simulink model "model_SCARA_comp_torque_joint_space"  (R2022b)
settings: Solver=VariableStepAuto  StartTime=0.0  StopTime=times_way(end)  RelTol=1e-3
undefined symbols (not defined in the file or in its folder): eta_des0, q1_0, q1_dot_0, q2_0, q2_dot_0, q3_0, q3_dot_0, q4_0, q4_dot_0
libraries: robotcorelib x1
settings Model: Creator=anton  LastModifiedBy=anton

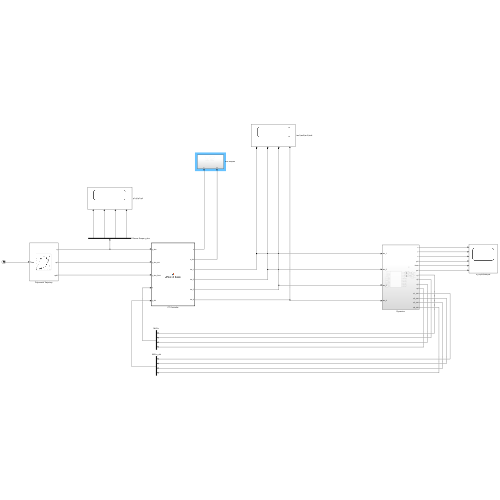
[thumbnail: Simulink's stored preview of the top-level diagram]
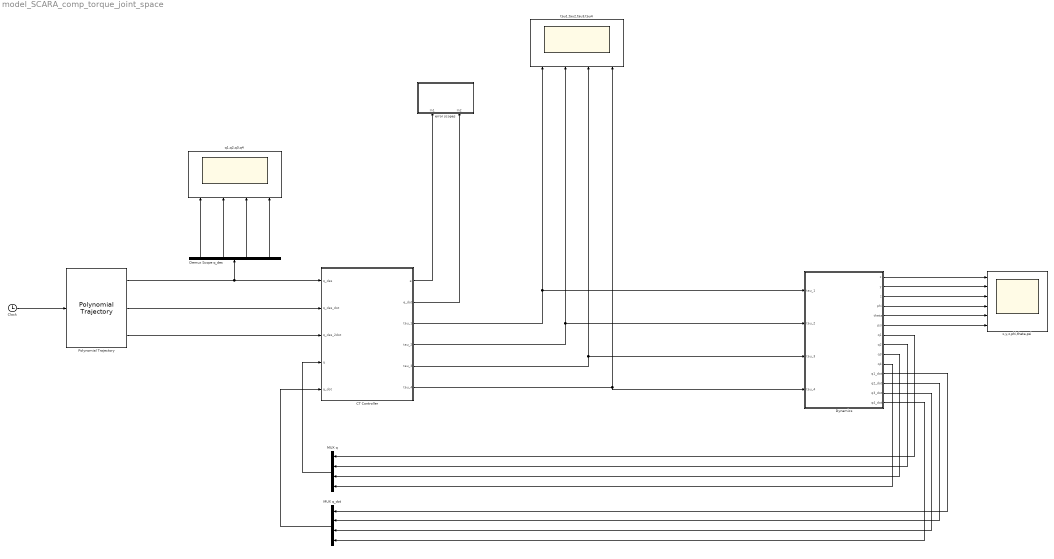
== system model_SCARA_comp_torque_joint_space ==
  CT Controller : MATLAB Function  TreatAsAtomicUnit=on
  Clock : Clock
  Demux Scope q_des : Demux
  Dynamics : Subsystem
  MUX q : Mux
  MUX q_dot : Mux
  Polynomial Trajectory : robotcorelib/Polynomial Trajectory  WaypointSource=Internal  Waypoints=waypoints  TimePoints=times_way  TimeInterval=times_way  Method=Cubic Polynomial  ParameterSource=Internal  VelocityBoundaryCondition=zeros(4,5)  AccelerationBoundaryCondition=zeros( 2, 5 )  SimulateUsing=Interpreted execution
  error scopes : Subsystem
  q1,q2,q3,q4 : Scope  NumInputPorts=4
  tau1,tau2,tau3,tau4 : Scope  NumInputPorts=4
  x,y,z,phi,theta,psi : Scope  NumInputPorts=6
  wires:
  Dynamics/7(q1) -> MUX q/1
  Dynamics/8(q2) -> MUX q/2
  Dynamics/9(q3) -> MUX q/3
  Dynamics/10(q4) -> MUX q/4
  Dynamics/11(q1_dot) -> MUX q_dot/1
  Dynamics/12(q2_dot) -> MUX q_dot/2
  Dynamics/13(q3_dot) -> MUX q_dot/3
  Dynamics/14(q4_dot) -> MUX q_dot/4
  MUX q/1 -> CT Controller/4(q)
  MUX q_dot/1 -> CT Controller/5(q_dot)
  Clock/1 -> Polynomial Trajectory/1
  Polynomial Trajectory/1 -> Demux Scope q_des/1, CT Controller/1(q_des)
  Demux Scope q_des/1 -> q1,q2,q3,q4/1
  Demux Scope q_des/2 -> q1,q2,q3,q4/2
  Demux Scope q_des/3 -> q1,q2,q3,q4/3
  Demux Scope q_des/4 -> q1,q2,q3,q4/4
  Dynamics/6(psi) -> x,y,z,phi,theta,psi/6
  Dynamics/1(x) -> x,y,z,phi,theta,psi/1
  Dynamics/2(y) -> x,y,z,phi,theta,psi/2
  Dynamics/3(z) -> x,y,z,phi,theta,psi/3
  Dynamics/4(phi) -> x,y,z,phi,theta,psi/4
  Dynamics/5(theta) -> x,y,z,phi,theta,psi/5
  CT Controller/6(tau_4) -> tau1,tau2,tau3,tau4/4, Dynamics/4(tau_4)
  CT Controller/5(tau_3) -> tau1,tau2,tau3,tau4/3, Dynamics/3(tau_3)
  CT Controller/4(tau_2) -> tau1,tau2,tau3,tau4/2, Dynamics/2(tau_2)
  CT Controller/3(tau_1) -> tau1,tau2,tau3,tau4/1, Dynamics/1(tau_1)
  Polynomial Trajectory/2 -> CT Controller/2(q_des_dot)
  Polynomial Trajectory/3 -> CT Controller/3(q_des_2dot)
  CT Controller/1(e) -> error scopes/1(In1)
  CT Controller/2(e_dot) -> error scopes/2(In2)

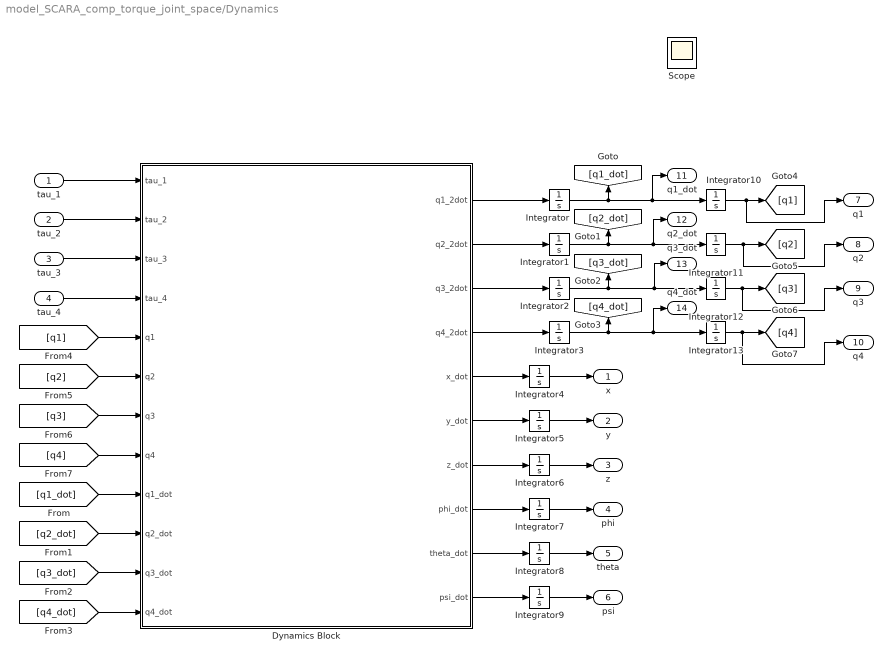
== system model_SCARA_comp_torque_joint_space/Dynamics ==
  tau_1 : Inport
  tau_2 : Inport  Port=2
  tau_3 : Inport  Port=3
  tau_4 : Inport  Port=4
  Dynamics Block : MATLAB Function  TreatAsAtomicUnit=on
  Integrator : Integrator  InitialCondition=q1_dot_0
  Integrator1 : Integrator  InitialCondition=q2_dot_0
  Integrator10 : Integrator  InitialCondition=q1_0  WrapState=on
  Integrator11 : Integrator  InitialCondition=q2_0  WrapState=on
  Integrator12 : Integrator  InitialCondition=q3_0  WrapState=on
  Integrator13 : Integrator  InitialCondition=q4_0
  Integrator2 : Integrator  InitialCondition=q3_dot_0
  Integrator3 : Integrator  InitialCondition=q4_dot_0
  Integrator4 : Integrator  InitialCondition=eta_des0(1)
  Integrator5 : Integrator  InitialCondition=eta_des0(2)
  Integrator6 : Integrator  InitialCondition=eta_des0(3)
  Integrator7 : Integrator
  Integrator8 : Integrator
  Integrator9 : Integrator  InitialCondition=eta_des0(4)  WrapState=on
  Scope : Scope  NumInputPorts=4
  x : Outport
  y : Outport  Port=2
  z : Outport  Port=3
  phi : Outport  Port=4
  theta : Outport  Port=5
  psi : Outport  Port=6
  q1 : Outport  Port=7
  q2 : Outport  Port=8
  q3 : Outport  Port=9
  q4 : Outport  Port=10
  q1_dot : Outport  Port=11
  q2_dot : Outport  Port=12
  q3_dot : Outport  Port=13
  q4_dot : Outport  Port=14
  wires:
  Dynamics Block/1(q1_2dot) -> Integrator/1
  Dynamics Block/2(q2_2dot) -> Integrator1/1
  Dynamics Block/3(q3_2dot) -> Integrator2/1
  Dynamics Block/4(q4_2dot) -> Integrator3/1
  Integrator/1 -> Integrator10/1, q1_dot/1, [q1_dot]
  [q1_dot] -> Dynamics Block/9(q1_dot)
  Integrator1/1 -> q2_dot/1, Integrator11/1, [q2_dot]
  Integrator2/1 -> q3_dot/1, Integrator12/1, [q3_dot]
  Integrator3/1 -> q4_dot/1, Integrator13/1, [q4_dot]
  [q2_dot] -> Dynamics Block/10(q2_dot)
  Integrator10/1 -> q1/1, [q1]
  Integrator11/1 -> q2/1, [q2]
  Integrator12/1 -> [q3], q3/1
  Integrator13/1 -> q4/1, [q4]
  [q3_dot] -> Dynamics Block/11(q3_dot)
  [q4_dot] -> Dynamics Block/12(q4_dot)
  [q1] -> Dynamics Block/5(q1)
  [q2] -> Dynamics Block/6(q2)
  [q3] -> Dynamics Block/7(q3)
  [q4] -> Dynamics Block/8(q4)
  tau_4/1 -> Dynamics Block/4(tau_4)
  tau_3/1 -> Dynamics Block/3(tau_3)
  tau_2/1 -> Dynamics Block/2(tau_2)
  tau_1/1 -> Dynamics Block/1(tau_1)
  Dynamics Block/8(phi_dot) -> Integrator7/1
  Dynamics Block/7(z_dot) -> Integrator6/1
  Dynamics Block/6(y_dot) -> Integrator5/1
  Dynamics Block/5(x_dot) -> Integrator4/1
  Integrator4/1 -> x/1
  Dynamics Block/9(theta_dot) -> Integrator8/1
  Dynamics Block/10(psi_dot) -> Integrator9/1
  Integrator5/1 -> y/1
  Integrator6/1 -> z/1
  Integrator7/1 -> phi/1
  Integrator8/1 -> theta/1
  Integrator9/1 -> psi/1

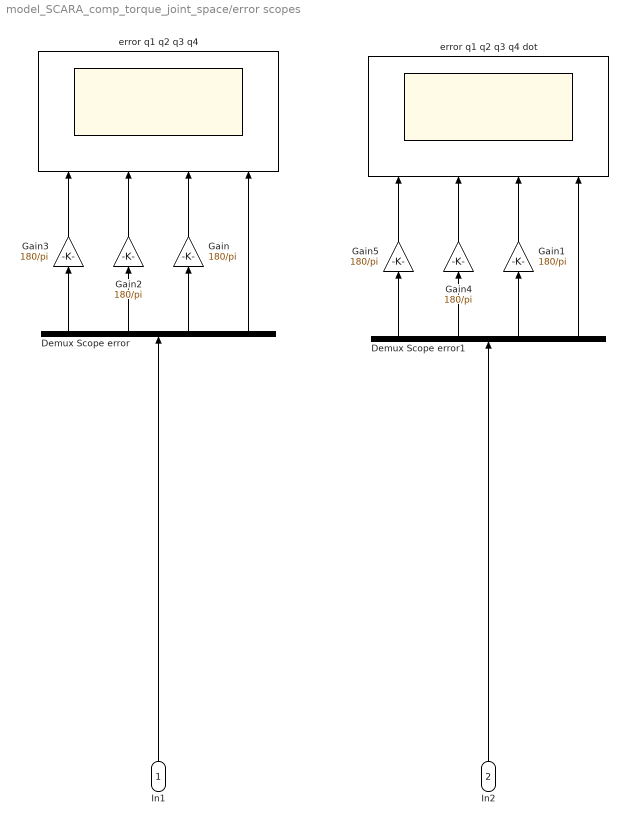
== system model_SCARA_comp_torque_joint_space/error scopes ==
  In1 : Inport
  In2 : Inport  Port=2
  Demux Scope error : Demux
  Demux Scope error1 : Demux
  Gain{,1..5} (6 alike) : Gain  Gain=180/pi
  error q1 q2 q3 q4 : Scope  NumInputPorts=4
  error q1 q2 q3 q4 dot : Scope  NumInputPorts=4
  wires:
  Gain1/1 -> error q1 q2 q3 q4 dot/3
  Demux Scope error/1 -> Gain3/1
  Gain/1 -> error q1 q2 q3 q4/3
  Demux Scope error/3 -> Gain/1
  Gain5/1 -> error q1 q2 q3 q4 dot/1
  In2/1 -> Demux Scope error1/1
  Demux Scope error1/4 -> error q1 q2 q3 q4 dot/4
  Gain2/1 -> error q1 q2 q3 q4/2
  Demux Scope error/2 -> Gain2/1
  Demux Scope error1/1 -> Gain5/1
  Demux Scope error1/2 -> Gain4/1
  In1/1 -> Demux Scope error/1
  Demux Scope error1/3 -> Gain1/1
  Demux Scope error/4 -> error q1 q2 q3 q4/4
  Gain4/1 -> error q1 q2 q3 q4 dot/2
  Gain3/1 -> error q1 q2 q3 q4/1

== matlab function model_SCARA_comp_torque_joint_space/CT Controller ==
  data: e output; e_dot output; q_des input size=[4 1]; q_des_dot input; q_des_2dot input; q input size=[4,1]; tau_1 output size=1; tau_2 output size=1; tau_3 output size=1; tau_4 output size=1; q_dot input size=[4,1]
function [e,e_dot,tau_1,tau_2,tau_3,tau_4] = Computed_Torque(q_des,q_des_dot,q_des_2dot, q,q_dot)
%% Parameters Definition

% masses

m1 = 20; % [kg]
m2 = 15; % [kg]
m3 = 15; % [kg]
m4 = 0.5; % [kg]

% link length

l0 = 0; % [m]
l1 = 0.2; % [m]
l2 = 0.25; % [m]
l_j1j2 = 0.02; % [m]

% lenght joint to COM

r1 = 0.1; % [m]
r2 = 0.125; % [m]

% inertia

Iz1 = 0.27; % [kg*m^2]
Iz2 = 0.31; % [kg*m^2]
Iz3 = 0.02; % [kg*m^2]
Iz4 = 0.0001; % [kg*m^2]

% gravity
g = 9.81; % [m/s^2]

q1_des = q_des(1);
q2_des = q_des(2);
q3_des = q_des(3);
q4_des = q_des(4);

q1_des_dot = q_des_dot(1);
q2_des_dot = q_des_dot(2);
q3_des_dot = q_des_dot(3);
q4_des_dot = q_des_dot(4);


q1_des_2dot = q_des_2dot(1);
q2_des_2dot = q_des_2dot(2);
q3_des_2dot = q_des_2dot(3);
q4_des_2dot = q_des_2dot(4);

q1 = q(1);
q2 = q(2);
q3 = q(3);
q4 = q(4);

q1_dot = q_dot(1);
q2_dot = q_dot(2);
q3_dot = q_dot(3);
q4_dot = q_dot(4);


% eta = [- l2*sin(q1 + q2) - l1*sin(q1); 
%         l2*cos(q1 + q2) + l1*cos(q1); 
%         l0 + q4; 
%         q1 + q2 + q3];
% 
% eta_des = [- l2*sin(q1_des + q2_des) - l1*sin(q1_des); 
%         l2*cos(q1_des + q2_des) + l1*cos(q1_des); 
%         l0 + q4_des; 
%         q1_des + q2_des + q3_des];
% 
% J = [-1/10, l1*cos(q1 + q2) - l1*cos(q2) - 1/8, l1*cos(q1 + q2 + q3) - l2*cos(q3) - l1*cos(q2 + q3) + l2*cos(q1 + q2 + q3), 0; 
%     0, -l1*(sin(q1 + q2) - sin(q2)), l1*sin(q2 + q3) + l2*sin(q3) - l1*sin(q1 + q2 + q3) - l2*sin(q1 + q2 + q3), 0; 
%     0, 0, 0, 1; 
%     1, 1, 1, 0];
% 
% %eta_dot = J*q_dot;
% 
% eta_dot = [- q1_dot/10 - q3_dot*(l1*cos(q2 + q3) + l2*cos(q3) - l1*cos(q1 + q2 + q3) - l2*cos(q1 + q2 + q3)) - q2_dot*(l1*cos(q2) - l1*cos(q1 + q2) + (1/8)); 
%     q3_dot*(l1*sin(q2 + q3) + l2*sin(q3) - l1*sin(q1 + q2 + q3) - l2*sin(q1 + q2 + q3)) - l1*q2_dot*(sin(q1 + q2) - sin(q2)); 
%     q4_dot;
%     q1_dot + q2_dot + q3_dot];
% 
% % eta_2_dot = [l1*q3_dot^2*sin(q2 + q3) - 0.125*q2_2dot - l1*q2_2dot*cos(q2) - l2*q3_2dot*cos(q3) - l1*q2_dot^2*sin(q1 + q2) - 0.1*q1_2dot + l1*q3_2dot*cos(q1 + q2 + q3) + l2*q3_2dot*cos(q1 + q2 + q3) + l1*q2_dot^2*sin(q2) + l2*q3_dot^2*sin(q3) - l1*q3_dot^2*sin(q1 + q2 + q3) - l2*q3_dot^2*sin(q1 + q2 + q3) + l1*q2_2dot*cos(q1 + q2) - l1*q3_2dot*cos(q2 + q3) - l1*q1_dot*q2_dot*sin(q1 + q2) + l1*q2_dot*q3_dot*sin(q2 + q3) - l1*q1_dot*q3_dot*sin(q1 + q2 + q3) - l1*q2_dot*q3_dot*sin(q1 + q2 + q3) - l2*q1_dot*q3_dot*sin(q1 + q2 + q3) - l2*q2_dot*q3_dot*sin(q1 + q2 + q3); 
% %     q3_2dot*(l1*sin(q2 + q3) + l2*sin(q3) - l1*sin(q1 + q2 + q3) - l2*sin(q1 + q2 + q3)) - q3_dot*(q2_dot*(l1*cos(q1 + q2 + q3) - l1*cos(q2 + q3) + l2*cos(q1 + q2 + q3)) - q3_dot*(l1*cos(q2 + q3) + l2*cos(q3) - l1*cos(q1 + q2 + q3) - l2*cos(q1 + q2 + q3)) + q1_dot*cos(q1 + q2 + q3)*(l1 + l2)) - l1*q2_dot*(q1_dot*cos(q1 + q2) + q2_dot*cos(q1 + q2) - q2_dot*cos(q2)) - l1*q2_2dot*(sin(q1 + q2) - sin(q2)); 
% %     q4_2dot;
% %     0;
% %     0;
% %     q1_2dot + q2_2dot + q3_2dot];
% 
% eta_des_dot = [- q1_des_dot/10 - q3_des_dot*(l1*cos(q2_des + q3_des) + l2*cos(q3_des) - l1*cos(q1_des + q2_des + q3_des) - l2*cos(q1_des + q2_des + q3_des)) - q2_des_dot*(l1*cos(q2_des) - l1*cos(q1_des + q2_des) + (1/8)); 
%     q3_des_dot*(l1*sin(q2_des + q3_des) + l2*sin(q3_des) - l1*sin(q1_des + q2_des + q3_des) - l2*sin(q1_des + q2_des + q3_des)) - l1*q2_des_dot*(sin(q1_des + q2_des) - sin(q2_des)); 
%     q4_dot;
%     q1_des_dot + q2_des_dot + q3_des_dot];
% 
% eta_des_2dot = [l1*q3_des_dot^2*sin(q2_des + q3_des) - 0.125*q2_des_2dot - l1*q2_des_2dot*cos(q2_des) - l2*q3_des_2dot*cos(q3_des) - l1*q2_des_dot^2*sin(q1_des + q2_des) - 0.1*q1_des_2dot + l1*q3_des_2dot*cos(q1_des + q2_des + q3_des) + l2*q3_des_2dot*cos(q1_des + q2_des + q3_des) + l1*q2_des_dot^2*sin(q2_des) + l2*q3_des_dot^2*sin(q3_des) - l1*q3_des_dot^2*sin(q1_des + q2_des + q3_des) - l2*q3_des_dot^2*sin(q1_des + q2_des + q3_des) + l1*q2_des_2dot*cos(q1_des + q2_des) - l1*q3_des_2dot*cos(q2_des + q3_des) - l1*q1_des_dot*q2_des_dot*sin(q1_des + q2_des) + l1*q2_des_dot*q3_des_dot*sin(q2_des + q3_des) - l1*q1_des_dot*q3_des_dot*sin(q1_des + q2_des + q3_des) - l1*q2_des_dot*q3_des_dot*sin(q1_des + q2_des + q3_des) - l2*q1_des_dot*q3_des_dot*sin(q1_des + q2_des + q3_des) - l2*q2_des_dot*q3_des_dot*sin(q1_des + q2_des + q3_des); 
%     q3_des_2dot*(l1*sin(q2_des + q3_des) + l2*sin(q3_des) - l1*sin(q1_des + q2_des + q3_des) - l2*sin(q1_des + q2_des + q3_des)) - q3_des_dot*(q2_des_dot*(l1*cos(q1_des + q2_des + q3_des) - l1*cos(q2_des + q3_des) + l2*cos(q1_des + q2_des + q3_des)) - q3_des_dot*(l1*cos(q2_des + q3_des) + l2*cos(q3_des) - l1*cos(q1_des + q2_des + q3_des) - l2*cos(q1_des + q2_des + q3_des)) + q1_des_dot*cos(q1_des + q2_des + q3_des)*(l1 + l2)) - l1*q2_des_dot*(q1_des_dot*cos(q1_des + q2_des) + q2_des_dot*cos(q1_des + q2_des) - q2_des_dot*cos(q2_des)) - l1*q2_des_2dot*(sin(q1_des + q2_des) - sin(q2_des));
%     q4_des_2dot; 
%     q1_des_2dot + q2_des_2dot + q3_des_2dot];
% 
% J_dot = [0, - q2_dot*(l1*sin(q1 + q2) - l1*sin(q2)) - l1*q1_dot*sin(q1 + q2), q3_dot*(l1*sin(q2 + q3) + l2*sin(q3) - l1*sin(q1 + q2 + q3) - l2*sin(q1 + q2 + q3)) - q1_dot*(l1*sin(q1 + q2 + q3) + l2*sin(q1 + q2 + q3)) - q2_dot*(l1*sin(q1 + q2 + q3) - l1*sin(q2 + q3) + l2*sin(q1 + q2 + q3)), 0; 
%     0, - l1*q2_dot*(cos(q1 + q2) - cos(q2)) - l1*q1_dot*cos(q1 + q2), q3_dot*(l1*cos(q2 + q3) + l2*cos(q3) - l1*cos(q1 + q2 + q3) - l2*cos(q1 + q2 + q3)) - q2_dot*(l1*cos(q1 + q2 + q3) - l1*cos(q2 + q3) + l2*cos(q1 + q2 + q3)) - q1_dot*(l1*cos(q1 + q2 + q3) + l2*cos(q1 + q2 + q3)), 0; 
%     0, 0, 0, 0; 
%     0, 0, 0, 0];

%% Parameters for Matrices

alpha = Iz1 + r1^2*m1 + l1^2*m2 + l1^2*m3 + l1^2*m4;
beta = Iz2 + Iz3 + Iz4 + l2^2*m3 + l2^2*m4 + m2*r2^2;
gamma = l1*l2*m3 + l1*l2*m4 + l1*m2*r2;
delta = Iz3 + Iz4;

%% Dynamic Matrices

M = [alpha + beta + 2*gamma*cos(q2), beta + gamma*cos(q2), delta, 0;
    beta + gamma*cos(q2),                   beta,          delta, 0;
            delta,                          delta,         delta, 0; 
            0,                              0,                0, m4];
inv_M = eye(size(M))/M;
C = [-gamma*sin(q2)*q2_dot, -gamma*sin(q2)*(q1_dot + q2_dot), 0, 0;
    gamma*sin(q2) * q1_dot,             0,                    0, 0;
            0,                          0,                    0, 0; 
            0,                          0,                    0, 0];

G = [0; 0; 0; m4*g];

% inv_J = pinv(J);
% 
% h = C*q_dot + G;
% 
% M_eta = inv_J'*M*inv_J
% 
% 
% h_eta = inv_J' * h - M_eta * J_dot*q_dot
% 
% error_eta = eta_des - eta;
% error_eta_dot = eta_des_dot - eta_dot;


% alpha = error_eta(4); % errore su psi
% if(alpha > 0)
%     if(alpha > 2*pi - alpha)
%         error_eta(4) = - (2*pi - alpha);
%     else
%         error_eta(4) = alpha;
%     end
% 
% else
%     alpha = -alpha;
%     if(alpha > 2*pi - alpha)
%         error_eta(4) =  2*pi - alpha;
%     else
%         error_eta(4) = -alpha;
%     end
% end

% controllo nello spazio dei giunti
e = q_des-q;
e_dot = q_des_dot-q_dot;

 
kp1 = 1;
kp2 = 1;
kp3 = 1;
kp4 = 1;

kv1 = 1;
kv2 = 1;
kv3 = 1;
kv4 = 1;

Kp = 100*diag([kp1, kp2, kp3, kp4]);
Kv = 10*diag([kv1, kv2, kv3, kv4]);
for i = 1:3
    alpha = e(i); % errore su psi
    if(alpha > 0)
        if(alpha > 2*pi - alpha)
            e(i) = - (2*pi - alpha);
        else
            e(i) = alpha;
        end
    
    else
        alpha = -alpha;
        if(alpha > 2*pi - alpha)
            e(i) =  2*pi - alpha;
        else
            e(i) = -alpha;
        end
    end
end
% 
% Fcf = M_eta * (eta_des_2dot + Kv*error_eta_dot + Kp*error_eta) + h_eta;

% tau = J' * Fcf;
tau = M*(q_des_2dot + Kv*e_dot + Kp*e) + C*q_dot + G;

tau_1 = tau(1);
tau_2 = tau(2);
tau_3 = tau(3);
tau_4 = tau(4);

end

== matlab function model_SCARA_comp_torque_joint_space/Dynamics/Dynamics Block ==
  data: q1_2dot output size=1; q2_2dot output size=1; q3_2dot output size=1; q4_2dot output size=1; tau_1 input size=1; tau_2 input size=1; tau_3 input size=1; tau_4 input size=1; q1 input size=1; q2 input size=1; q3 input size=1; q4 input size=1; q1_dot input size=1; q2_dot input size=1; q3_dot input size=1; q4_dot input size=1; x_dot output; y_dot output; z_dot output; phi_dot output; theta_dot output; psi_dot output
function [q1_2dot, q2_2dot, q3_2dot, q4_2dot, x_dot,y_dot,z_dot,phi_dot,theta_dot,psi_dot] = Dynamics(tau_1,tau_2,tau_3,tau_4, q1,q2,q3,q4,q1_dot,q2_dot,q3_dot,q4_dot)

% Dynamic Model --> tau = M(q)*q_2dot + C(q,q_dot)*q_dot + G(q)
%
%% Parameters Definition

% masses

m1 = 20; % [kg]
m2 = 15; % [kg]
m3 = 15; % [kg]
m4 = 0.5; % [kg]

% link length

l0 = 0; % [m]
l1 = 0.2; % [m]
l2 = 0.25; % [m]

% lenght joint to COM

r1 = 0.1; % [m]
r2 = 0.125; % [m]

% inertia

Iz1 = 0.27; % [kg*m^2]
Iz2 = 0.31; % [kg*m^2]
Iz3 = 0.02; % [kg*m^2]
Iz4 = 0.0001; % [kg*m^2]

% gravity
g = 9.81; % [m/s^2]

%% Parameters for Matrices

alpha = Iz1 + r1^2*m1 + l1^2*m2 + l1^2*m3 + l1^2*m4;
beta = Iz2 + Iz3 + Iz4 + l2^2*m3 + l2^2*m4 + m2*r2^2;
gamma = l1*l2*m3 + l1*l2*m4 + l1*m2*r2;
delta = Iz3 + Iz4;

%% Dynamic Matrices

M = [alpha + beta + 2*gamma*cos(q2), beta + gamma*cos(q2), delta, 0;
    beta + gamma*cos(q2),                   beta,          delta, 0;
            delta,                          delta,         delta, 0; 
            0,                              0,                0, m4];

M_inv = eye(size(M))/M;

C = [-gamma*sin(q2)*q2_dot, -gamma*sin(q2)*(q1_dot + q2_dot), 0, 0;
    gamma*sin(q2) * q1_dot,             0,                    0, 0;
            0,                          0,                    0, 0; 
            0,                          0,                    0, 0];

G = [0; 0; 0; m4*g];

J = [- l2*cos(q1 + q2) - l1*cos(q1), -l2*cos(q1 + q2), (0), (0);
            - l2*sin(q1 + q2) - l1*sin(q1), -l2*sin(q1 + q2), (0), (0);
            (0), (0), (0), (1);
            0,0,0,0;
            0,0,0,0;
            (1), (1), (1), (0)];

% eta = [- l2*sin(q1 + q2) - l1*sin(q1); 
%     l2*cos(q1 + q2) + l1*cos(q1); 
%     l0 + q4; 
%     0;
%     0;
%     wrapToPi(q1 + q2 + q3)];
% 

%% Dynamics

q_dot = [q1_dot, q2_dot, q3_dot, q4_dot]';

tau = [tau_1, tau_2, tau_3, tau_4]';

% joint variable dynamics
q_2dot = M_inv*(tau - C*q_dot - G);

q1_2dot = q_2dot(1);
q2_2dot = q_2dot(2);
q3_2dot = q_2dot(3);
q4_2dot = q_2dot(4);


eta_dot = J*q_dot;

x_dot = eta_dot(1);
y_dot = eta_dot(2);
z_dot = eta_dot(3);
phi_dot = eta_dot(4);
theta_dot = eta_dot(5);
psi_dot = eta_dot(6);

% x = eta(1);
% y = eta(2);
% z = eta(3);
% phi = eta(4);
% theta = eta(5);
% psi = eta(6);

end
